simulink model "test"  (R2015a)
settings: Solver=ode45  StartTime=0.0  StopTime=10.0  RelTol=1e-3
undefined symbols (not defined in the file or in its folder): sineWave
settings Model: Creator=John  LastModifiedBy=John

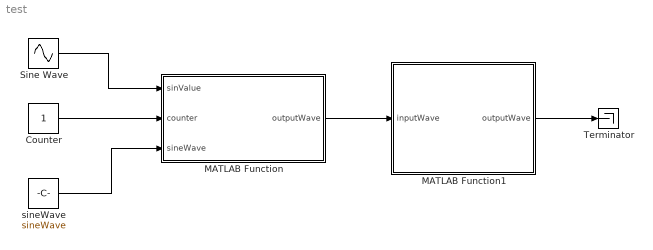
== system test ==
  Counter : Constant
  MATLAB Function : MATLAB Function  TreatAsAtomicUnit=on
  MATLAB Function1 : MATLAB Function  TreatAsAtomicUnit=on
  Sine Wave : Sin  Amplitude=2  SampleTime=0
  Terminator : Terminator
  sineWave : Constant  Value=sineWave
  wires:
  Sine Wave/1 -> MATLAB Function/1(sinValue)
  Counter/1 -> MATLAB Function/2(counter)
  MATLAB Function1/1(outputWave) -> Terminator/1
  MATLAB Function/1(outputWave) -> MATLAB Function1/1(inputWave)
  sineWave/1 -> MATLAB Function/3(sineWave)

== matlab function test/MATLAB Function1 ==
  data: inputWave input; outputWave output
function outputWave = sinHandler(inputWave)
%#codegen

outputWave = inputWave;

== matlab function test/MATLAB Function ==
  data: sinValue input; outputWave output; counter input; sineWave input
function outputWave = test(sinValue,counter,sineWave)
%function sineWave = test(sinValue,counter,sineWave)
load('SineData');
sineWave(counter) = sinValue;
counter = counter + 1;
save('SineData');
outputWave = sineWave;
end
